simulink model "projjfinal"  (R2022b)
settings: Solver=VariableStepAuto  StartTime=0.0  StopTime=10.0  RelTol=1e-3
undefined symbols (not defined in the file or in its folder): fraction, g, I, L, M, m, Muu
settings Model: Creator=HP  LastModifiedBy=HP

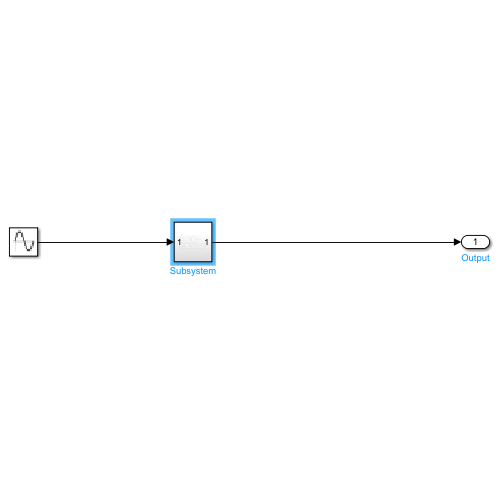
[thumbnail: Simulink's stored preview of the top-level diagram]
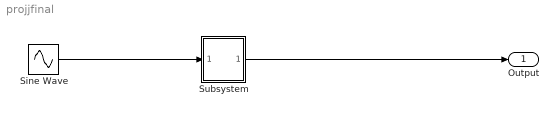
== system projjfinal ==
  Sine Wave : Sin  SampleTime=0
  Subsystem : Subsystem
  Output : Outport
  wires:
  Subsystem/1(Out1) -> Output/1
  Sine Wave/1 -> Subsystem/1(In1)

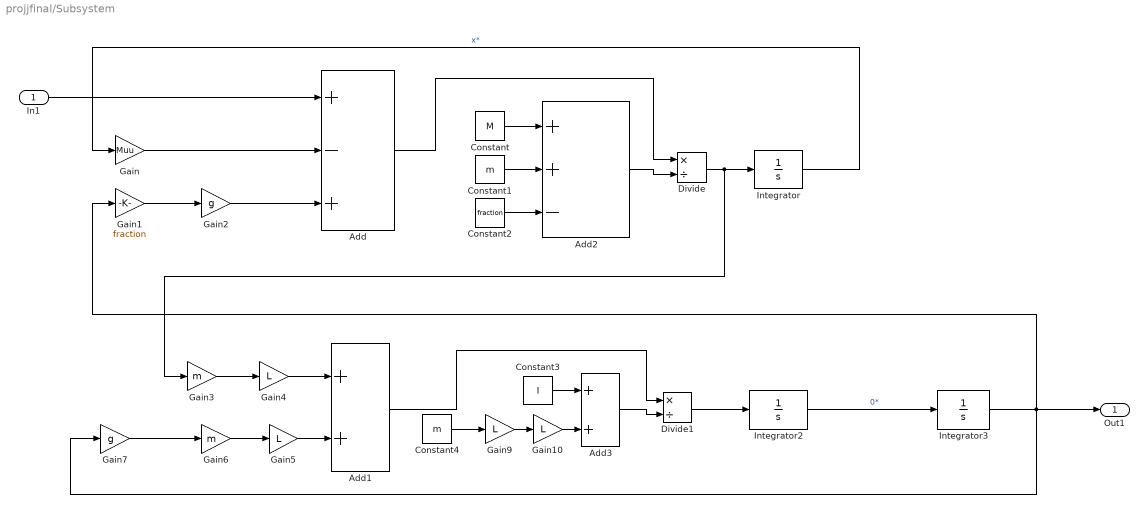
== system projjfinal/Subsystem ==
  In1 : Inport
  Add : Sum  Inputs=+-+
  Add1 : Sum
  Add2 : Sum  Inputs=++-
  Add3 : Sum
  Constant : Constant  Value=M
  Constant1 : Constant  Value=m
  Constant2 : Constant  Value=fraction
  Constant3 : Constant  Value=I
  Constant4 : Constant  Value=m
  Divide : Product  Inputs=*/
  Divide1 : Product  Inputs=*/
  Gain : Gain  Gain=Muu
  Gain1 : Gain  Gain=fraction
  Gain{4..5,9..10} (4 alike) : Gain  Gain=L
  Gain2 : Gain  Gain=g
  Gain3 : Gain  Gain=m
  Gain6 : Gain  Gain=m
  Gain7 : Gain  Gain=g
  Integrator : Integrator
  Integrator2 : Integrator
  Integrator3 : Integrator
  Out1 : Outport
  wires:
  Constant4/1 -> Gain9/1
  Constant1/1 -> Add2/2
  Integrator3/1 -> Gain7/1, Out1/1, Gain1/1
  Constant/1 -> Add2/1
  Gain6/1 -> Gain5/1
  Gain7/1 -> Gain6/1
  Gain/1 -> Add/2
  Divide/1 -> Gain3/1, Integrator/1
  Gain1/1 -> Gain2/1
  Constant2/1 -> Add2/3
  Gain10/1 -> Add3/2
  Gain2/1 -> Add/3
  Integrator/1 -> Gain/1  "x*"
  Integrator2/1 -> Integrator3/1  "0*"
  Gain3/1 -> Gain4/1
  Gain5/1 -> Add1/2
  Add/1 -> Divide/1
  In1/1 -> Add/1
  Constant3/1 -> Add3/1
  Gain9/1 -> Gain10/1
  Add2/1 -> Divide/2
  Add1/1 -> Divide1/1
  Add3/1 -> Divide1/2
  Gain4/1 -> Add1/1
  Divide1/1 -> Integrator2/1
